simulink model "gm_SG"  (R2019a)
settings: Solver=FixedStepDiscrete  StartTime=0.0  StopTime=stop_time  RelTol=1e-3
InitFcn:
  | SG_callback_init
StopFcn:
  | SG_callback_stop
undefined symbols (not defined in the file or in its folder): Ts_system
libraries: simulink x3
settings Model: Creator=Ross  LastModifiedBy=Ross
settings DataIOCC: ReturnWorkspaceOutputs=off
settings OptimizationCC: BlockReduction=off  ConditionallyExecuteInputs=off  DefaultParameterBehavior=Inlined
settings DebuggingCC: ReadBeforeWriteMsg=DisableAll  WriteAfterWriteMsg=DisableAll  WriteAfterReadMsg=DisableAll  AlgebraicLoopMsg=error  InheritedTsInSrcMsg=none  MultiTaskDSMMsg=none  SingleTaskRateTransMsg=error  PregeneratedLibrarySubsystemCodeDiagnostic=none  ArithmeticOperatorsInVariantConditions=warning
settings HardwareCC: ProdBitPerPointer=32  ProdBitPerSizeT=32  ProdBitPerPtrDiffT=32  ProdLargestAtomicFloat=None  ProdIntDivRoundTo=Undefined  ProdEndianess=Unspecified  ProdWordSize=32  ProdHWDeviceType=ASIC/FPGA->ASIC/FPGA  TargetBitPerPointer=64  TargetBitPerSizeT=64  TargetBitPerPtrDiffT=64  TargetLongLongMode=on  TargetIntDivRoundTo=Zero  TargetEndianess=LittleEndian  TargetWordSize=64  TargetHWDeviceType=Custom Processor->MATLAB Host Computer  ProdEqTarget=off
settings ModelReferenceCC: UpdateModelReferenceTargets=IfOutOfDate
settings SFSimCC: SFSimEcho=off  SimUseLocalCustomCode=off
settings RTWCC: RTWUseLocalCustomCode=off

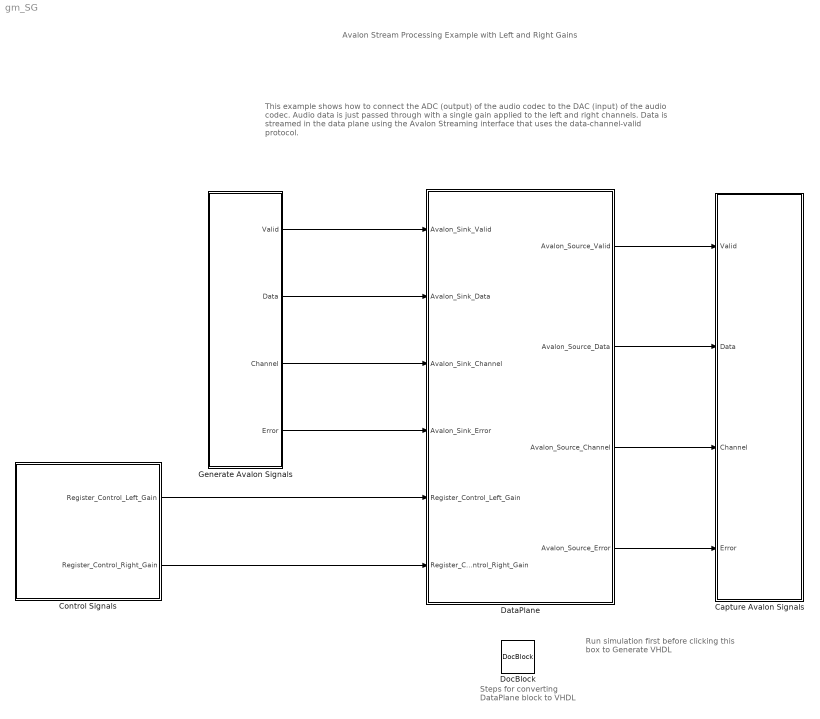
== system gm_SG ==
  note: Run simulation first
      | before clicking this box to
      | Generate VHDL
  note: Avalon Stream Processing Example
      | with Left and Right Gains
  note: Steps for converting
      | DataPlane block
      | to VHDL
  note: This example shows how to connect the ADC (output) of the audio codec to the DAC (input) of the audio codec. Audio data is just passed through with a single gain applied to the left and right channels. Data is streamed in the data plane using the Avalon Streaming interface that uses the data-channel-valid protocol.
  Capture Avalon Signals : Subsystem
  Control Signals : Subsystem
  DataPlane : Subsystem  TreatAsAtomicUnit=on
  DocBlock : simulink/Model-Wide Utilities/DocBlock  DocumentType=HTML
  Generate Avalon Signals : Subsystem
  wires:
  Control Signals/2(Register_Control_Right_Gain) -> DataPlane/6(Register_Control_Right_Gain)
  Control Signals/1(Register_Control_Left_Gain) -> DataPlane/5(Register_Control_Left_Gain)
  DataPlane/4(Avalon_Source_Error) -> Capture Avalon Signals/4(Error)
  DataPlane/3(Avalon_Source_Channel) -> Capture Avalon Signals/3(Channel)
  DataPlane/1(Avalon_Source_Valid) -> Capture Avalon Signals/1(Valid)
  DataPlane/2(Avalon_Source_Data) -> Capture Avalon Signals/2(Data)
  Generate Avalon Signals/4(Error) -> DataPlane/4(Avalon_Sink_Error)
  Generate Avalon Signals/3(Channel) -> DataPlane/3(Avalon_Sink_Channel)
  Generate Avalon Signals/1(Valid) -> DataPlane/1(Avalon_Sink_Valid)
  Generate Avalon Signals/2(Data) -> DataPlane/2(Avalon_Sink_Data)

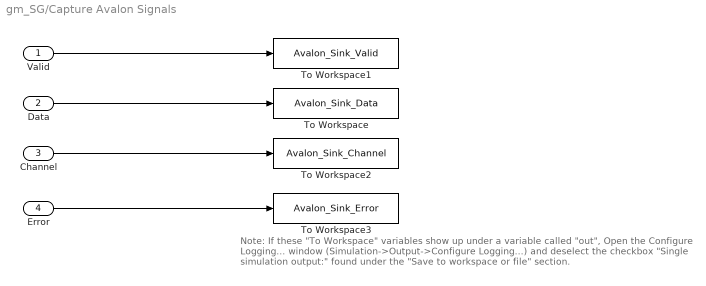
== system gm_SG/Capture Avalon Signals ==
  note: Note:  If these "To Workspace" variables show up under a variable called "out",
      | Open the Configure Logging... window (Simulation->Output->Configure Logging...)
      | and deselect the checkbox "Single simulation output:" found under the "Save to workspace or file" section.
  Valid : Inport
  Data : Inport  Port=2
  Channel : Inport  Port=3
  Error : Inport  Port=4
  To Workspace : ToWorkspace  VariableName=Avalon_Sink_Data  SaveFormat=Timeseries  SampleTime=-1
  To Workspace1 : ToWorkspace  VariableName=Avalon_Sink_Valid  SaveFormat=Timeseries  SampleTime=-1
  To Workspace2 : ToWorkspace  VariableName=Avalon_Sink_Channel  SaveFormat=Timeseries  SampleTime=-1
  To Workspace3 : ToWorkspace  VariableName=Avalon_Sink_Error  SaveFormat=Timeseries  SampleTime=-1
  wires:
  Channel/1 -> To Workspace2/1
  Error/1 -> To Workspace3/1
  Valid/1 -> To Workspace1/1
  Data/1 -> To Workspace/1

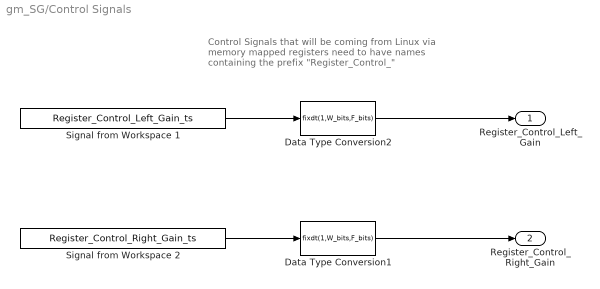
== system gm_SG/Control Signals ==
  note: Control Signals that will be coming from Linux via
      | memory mapped registers need to have names
      | containing the prefix "Register_Control_"
  Data Type Conversion1 : DataTypeConversion  OutDataTypeStr=fixdt(1,W_bits,F_bits)
  Data Type Conversion2 : DataTypeConversion  OutDataTypeStr=fixdt(1,W_bits,F_bits)
  Signal from Workspace 1 : FromWorkspace  VariableName=Register_Control_Left_Gain_ts  OutDataTypeStr=double  SampleTime=Ts_system
  Signal from Workspace 2 : FromWorkspace  VariableName=Register_Control_Right_Gain_ts  OutDataTypeStr=double  SampleTime=Ts_system
  Register_Control_Left_Gain : Outport
  Register_Control_Right_Gain : Outport  Port=2
  wires:
  Data Type Conversion1/1 -> Register_Control_Right_Gain/1
  Data Type Conversion2/1 -> Register_Control_Left_Gain/1
  Signal from Workspace 2/1 -> Data Type Conversion1/1
  Signal from Workspace 1/1 -> Data Type Conversion2/1

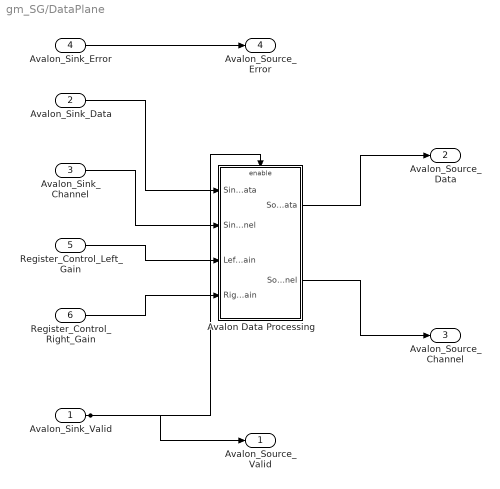
== system gm_SG/DataPlane ==
  Avalon_Sink_Valid : Inport  OutDataTypeStr=boolean  PortDimensions=1  SampleTime=2.03450520833333e-08
  Avalon_Sink_Data : Inport  Port=2  OutDataTypeStr=fixdt(1, 32, 28)  PortDimensions=1  SampleTime=2.03450520833333e-08
  Avalon_Sink_Channel : Inport  Port=3  OutDataTypeStr=fixdt(0, 2, 0)  PortDimensions=1  SampleTime=2.03450520833333e-08
  Avalon_Sink_Error : Inport  Port=4  OutDataTypeStr=fixdt(0, 2, 0)  PortDimensions=1  SampleTime=2.03450520833333e-08
  Register_Control_Left_Gain : Inport  Port=5  OutDataTypeStr=fixdt(1, 32, 28)  PortDimensions=1  SampleTime=2.03450520833333e-08
  Register_Control_Right_Gain : Inport  Port=6  OutDataTypeStr=fixdt(1, 32, 28)  PortDimensions=1  SampleTime=2.03450520833333e-08
  Avalon Data Processing : Subsystem
  Avalon_Source_Valid : Outport
  Avalon_Source_Data : Outport  Port=2
  Avalon_Source_Channel : Outport  Port=3
  Avalon_Source_Error : Outport  Port=4
  wires:
  Avalon_Sink_Valid/1 -> Avalon_Source_Valid/1, Avalon Data Processing/Enable
  Avalon_Sink_Data/1 -> Avalon Data Processing/1(Sink_Data)
  Avalon_Sink_Channel/1 -> Avalon Data Processing/2(Sink_Channel)
  Avalon_Sink_Error/1 -> Avalon_Source_Error/1
  Register_Control_Left_Gain/1 -> Avalon Data Processing/3(Left_Gain)
  Register_Control_Right_Gain/1 -> Avalon Data Processing/4(Right_Gain)
  Avalon Data Processing/1(Source_Data) -> Avalon_Source_Data/1
  Avalon Data Processing/2(Source_Channel) -> Avalon_Source_Channel/1

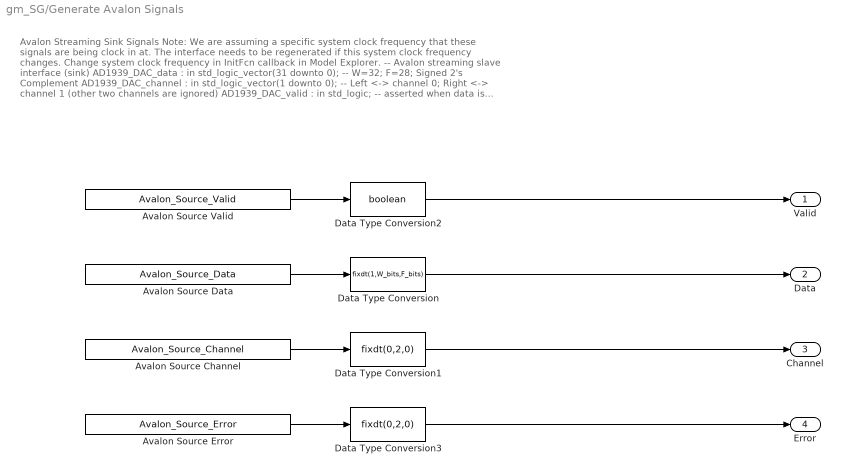
== system gm_SG/Generate Avalon Signals ==
  note: Avalon Streaming Sink Signals
      | Note: We are assuming a specific system clock frequency that these signals are being clock in at.
      | The interface needs to be regenerated if this system clock frequency changes. Change system clock frequency in InitFcn callback in Model Explorer.
      |
      | -- Avalon streaming slave interface (sink)
      | AD1939_DAC_data : in std_logic_vector(31 downto 0); -- W=32; F=28; Signed 2's Complement
      | AD1939_DAC_channel : in std_logic_vector(1 downto 0); -- Left <-> channel 0; Right <-> channel 1 (other two channels are ignored)
      | AD1939_DAC_valid : in std_logic; -- asserted when data is valid
      | AD1939_DAC_error : in std_logic_vector(1 downto 0) -- error channel is ignored, assumed to be error free at this point
      |
      | For more information on the data-channel-valid protocol, s ee chapter 5 in Intel's Avalon Interfaced Specification (p. 40) at https://www.intel.com/content/dam/www/programmable/us/en/pdfs/literature/manual/mnl_avalon_spec.pdf
  Avalon Source Channel : FromWorkspace  VariableName=Avalon_Source_Channel  OutDataTypeStr=double  SampleTime=Ts_system
  "Avalon Source Data " : FromWorkspace  VariableName=Avalon_Source_Data  OutDataTypeStr=double  SampleTime=Ts_system
  Avalon Source Error : FromWorkspace  VariableName=Avalon_Source_Error  OutDataTypeStr=double  SampleTime=Ts_system
  Avalon Source Valid : FromWorkspace  VariableName=Avalon_Source_Valid  OutDataTypeStr=double  SampleTime=Ts_system
  Data Type Conversion : DataTypeConversion  OutDataTypeStr=fixdt(1,W_bits,F_bits)
  Data Type Conversion1 : DataTypeConversion  OutDataTypeStr=fixdt(0,2,0)
  Data Type Conversion2 : DataTypeConversion  OutDataTypeStr=boolean
  Data Type Conversion3 : DataTypeConversion  OutDataTypeStr=fixdt(0,2,0)
  Valid : Outport
  Data : Outport  Port=2
  Channel : Outport  Port=3
  Error : Outport  Port=4
  wires:
  "Avalon Source Data "/1 -> Data Type Conversion/1
  Avalon Source Channel/1 -> Data Type Conversion1/1
  Data Type Conversion3/1 -> Error/1
  Avalon Source Valid/1 -> Data Type Conversion2/1
  Data Type Conversion/1 -> Data/1
  Avalon Source Error/1 -> Data Type Conversion3/1
  Data Type Conversion2/1 -> Valid/1
  Data Type Conversion1/1 -> Channel/1

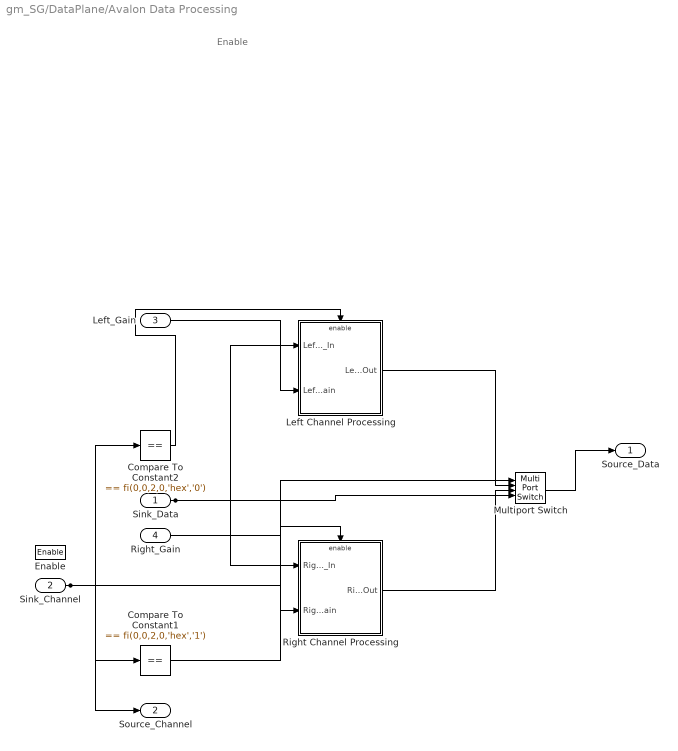
== system gm_SG/DataPlane/Avalon Data Processing ==
  note: Enable
  Sink_Data : Inport  OutDataTypeStr=fixdt(1, 32, 28)  PortDimensions=1  SampleTime=2.03450520833333e-08
  Sink_Channel : Inport  Port=2  OutDataTypeStr=fixdt(0, 2, 0)  PortDimensions=1  SampleTime=2.03450520833333e-08
  Left_Gain : Inport  Port=3  OutDataTypeStr=fixdt(1, 32, 28)  PortDimensions=1  SampleTime=2.03450520833333e-08
  Right_Gain : Inport  Port=4  OutDataTypeStr=fixdt(1, 32, 28)  PortDimensions=1  SampleTime=2.03450520833333e-08
  Enable : EnablePort  OutDataTypeStr=boolean
  Compare To Constant1 : simulink/Logic and Bit Operations/Compare To Constant  relop===  const=fi(0,0,2,0,'hex','1')  OutDataTypeStr=boolean
  Compare To Constant2 : simulink/Logic and Bit Operations/Compare To Constant  relop===  const=fi(0,0,2,0,'hex','0')  OutDataTypeStr=boolean
  Left Channel Processing : Subsystem
  Multiport Switch : MultiPortSwitch  DataPortOrder=Zero-based contiguous  DiagnosticForDefault=None  zeroidx=on  OutDataTypeStr=fixdt(1, 32, 28)  SampleTime=2.03450520833333e-08
  Right Channel Processing : Subsystem
  Source_Data : Outport  InitialOutput=0
  Source_Channel : Outport  Port=2  InitialOutput=0
  wires:
  Sink_Data/1 -> Multiport Switch/4, Right Channel Processing/1(Right_Data_In), Left Channel Processing/1(Left_Data_In)
  Sink_Channel/1 -> Multiport Switch/1, Compare To Constant2/1, Compare To Constant1/1, Source_Channel/1
  Left_Gain/1 -> Left Channel Processing/2(Left_Gain)
  Right_Gain/1 -> Right Channel Processing/2(Right_Gain)
  Compare To Constant1/1 -> Right Channel Processing/Enable
  Compare To Constant2/1 -> Left Channel Processing/Enable
  Left Channel Processing/1("Left_Data_Out ") -> Multiport Switch/2
  Multiport Switch/1 -> Source_Data/1
  Right Channel Processing/1("Right_Data_Out ") -> Multiport Switch/3

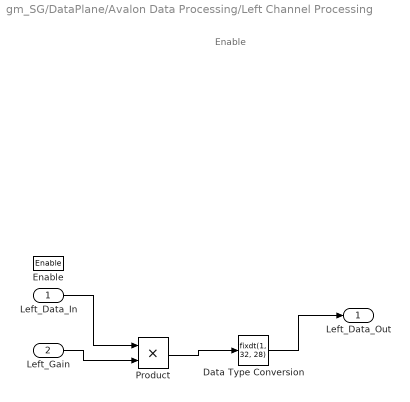
== system gm_SG/DataPlane/Avalon Data Processing/Left Channel Processing ==
  note: Enable
  Left_Data_In : Inport  OutDataTypeStr=fixdt(1, 32, 28)  PortDimensions=1  SampleTime=2.03450520833333e-08
  Left_Gain : Inport  Port=2  OutDataTypeStr=fixdt(1, 32, 28)  PortDimensions=1  SampleTime=2.03450520833333e-08
  Enable : EnablePort  OutDataTypeStr=boolean
  Data Type Conversion : DataTypeConversion  OutDataTypeStr=fixdt(1, 32, 28)  SampleTime=2.03450520833333e-08
  Product : Product  Inputs=**  OutDataTypeStr=fixdt(1, 64, 56)  SampleTime=2.03450520833333e-08
  "Left_Data_Out " : Outport  InitialOutput=0
  wires:
  Left_Data_In/1 -> Product/1
  Left_Gain/1 -> Product/2
  Data Type Conversion/1 -> "Left_Data_Out "/1
  Product/1 -> Data Type Conversion/1

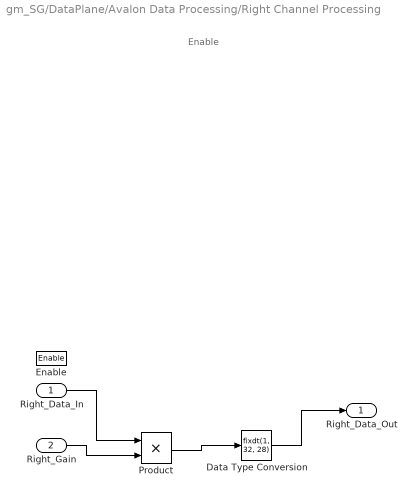
== system gm_SG/DataPlane/Avalon Data Processing/Right Channel Processing ==
  note: Enable
  Right_Data_In : Inport  OutDataTypeStr=fixdt(1, 32, 28)  PortDimensions=1  SampleTime=2.03450520833333e-08
  Right_Gain : Inport  Port=2  OutDataTypeStr=fixdt(1, 32, 28)  PortDimensions=1  SampleTime=2.03450520833333e-08
  Enable : EnablePort  OutDataTypeStr=boolean
  Data Type Conversion : DataTypeConversion  OutDataTypeStr=fixdt(1, 32, 28)  SampleTime=2.03450520833333e-08
  Product : Product  Inputs=**  OutDataTypeStr=fixdt(1, 64, 56)  SampleTime=2.03450520833333e-08
  "Right_Data_Out " : Outport  InitialOutput=0
  wires:
  Right_Data_In/1 -> Product/1
  Right_Gain/1 -> Product/2
  Data Type Conversion/1 -> "Right_Data_Out "/1
  Product/1 -> Data Type Conversion/1
